simulink model "HelloWorldCont"  (Simulink 7.1)
settings: Solver=ode1  StartTime=0.0  StopTime=30  FixedStep=1  MaxStep=1  RelTol=1e-3
undefined symbols (not defined in the file or in its folder): uk, xk
libraries: MPCMdlLib x9
settings Model: Creator=vichik  LastModifiedBy=serg

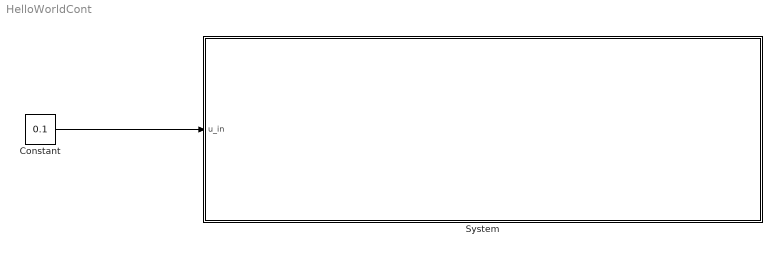
== system HelloWorldCont ==
  Constant : Constant  Value=0.1
  System : Subsystem
  wires:
  Constant/1 -> System/1(u_in)

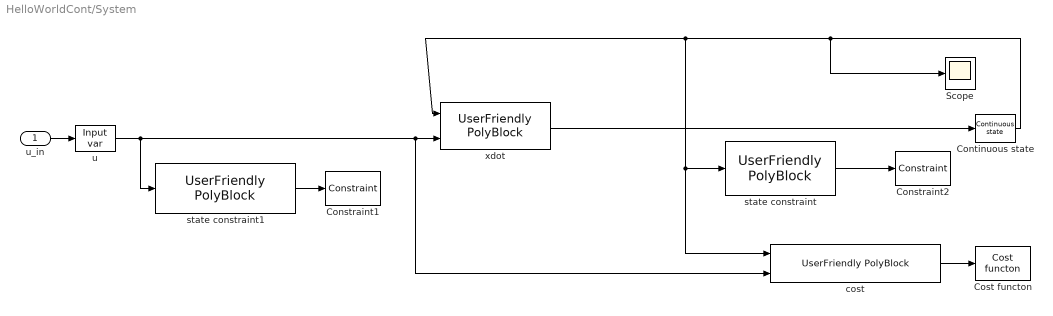
== system HelloWorldCont/System ==
  u_in : Inport
  Constraint1 : MPCMdlLib/Constraint  Tag=InequalBlock  CompareSign=< 0
  Constraint2 : MPCMdlLib/Constraint  Tag=InequalBlock  CompareSign=< 0
  Continuous state : MPCMdlLib/Continuous state  Tag=OptState  SystemSampleTime=-1  init_val=0.6  save_name=BL_System_Continuous_state
  Cost functon : MPCMdlLib/Cost functon  Tag=OptCost
  Scope : Scope
  "cost " : MPCMdlLib/UserFriendly PolyBlock  Tag=PolyBlock  A=[2 0; 0 2]  C=[0.5 2]  gA=[0 0 ]  gC=1  input_type=Scalar  output_type=Scalar  port_names=xk,uk
  state constraint : MPCMdlLib/UserFriendly PolyBlock  Tag=PolyBlock  A="[1  ;  0 ]"  C=[1 -1 ; -1 0.5 ]  gA="[0  ]"  gC=1  input_type=Scalar  output_type=Vector  port_names=x
  state constraint1 : MPCMdlLib/UserFriendly PolyBlock  Tag=PolyBlock  A="[1  ;  0 ]"  C=[1 -2 ; -1 -2 ]  gA="[0  ]"  gC=1  input_type=Scalar  output_type=Vector  port_names=u
  u : MPCMdlLib/Input var  Tag=OptInput  SystemSampleTime=-1  step_ratio=1  save_name=BL_System_u
  xdot : MPCMdlLib/UserFriendly PolyBlock  Tag=PolyBlock  A=[1 0; 0 1]  C=[-0.1 1]  gA=[0 0 ]  gC=1  input_type=Scalar  output_type=Scalar  port_names=xk,uk
  wires:
  xdot/1 -> Continuous state/1
  Continuous state/1 -> xdot/1, state constraint/1, "cost "/1, Scope/1
  u/1 -> xdot/2, "cost "/2, state constraint1/1
  "cost "/1 -> Cost functon/1
  state constraint/1 -> Constraint2/1
  u_in/1 -> u/1
  state constraint1/1 -> Constraint1/1
